simulink model "ACC_Model"  (Simulink 7.6)
settings: Solver=ode5  StartTime=0.0  StopTime=inf  FixedStep=1/100  RelTol=1e-3
undefined symbols (not defined in the file or in its folder): DiscIntNeverNeededParam
libraries: simulink x21, simulink_extras x6
(part 3 of 4)

== system ACC_Model/ACC_System/TIS2 Bend Road/TIS2 Sorting Fun ==
  note: === TIS1 Sorting Fun block ===
      |
      |  - transforms information from the first sensor
      |    to the more appropriate form.
  TIS2range [m] : Inport
  TIS2rangedot [m/s] : Inport  Port=2
  TIS2theta [deg] : Inport  Port=3
  Degrees to Radians : simulink_extras/Transformations/Degrees to Radians  SystemSampleTime=-1
  Switch : Switch  Criteria=u2 ~= 0
  Unary Minus : UnaryMinus
  Unary Minus1 : UnaryMinus
  range max : Constant  Value=5*TISMaxRange(2)
  TIS2_RANGE [m] : Outport
  TIS2_RANGEDOT [m/s] : Outport  Port=2
  TIS2_THETA [rad] : Outport  Port=3
  wires:
  Unary Minus/1 -> Degrees to Radians/1
  Switch/1 -> TIS2_RANGE [m]/1
  TIS2rangedot [m/s]/1 -> Unary Minus1/1
  range max/1 -> Switch/3
  Degrees to Radians/1 -> TIS2_THETA [rad]/1
  TIS2range [m]/1 -> Switch/2, Switch/1
  TIS2theta [deg]/1 -> Unary Minus/1
  Unary Minus1/1 -> TIS2_RANGEDOT [m/s]/1

== system ACC_Model/ACC_System/TIS2 Straight Road/Hold ==
  HWTflagIN : Inport
  lead_vel_in : Inport  Port=2
  HWTflagIN1 : InportShadow  Port=1
  If : If  IfExpression=u1 < 0.1  SampleTime=Tsensor
  If Action Subsystem : Subsystem  TreatAsAtomicUnit=on
  If Action Subsystem1 : Subsystem  TreatAsAtomicUnit=on
  Merge : Merge
  HWT_flag : Outport
  wires:
  lead_vel_in/1 -> If/1
  If/1 -> If Action Subsystem/Action
  If/2 -> If Action Subsystem1/Action
  If Action Subsystem/1(Out1) -> Merge/1
  If Action Subsystem1/1(Out1) -> Merge/2
  Merge/1 -> HWT_flag/1
  HWTflagIN/1 -> If Action Subsystem1/1(In1)
  HWTflagIN1/1 -> If Action Subsystem/1(In1)

== system ACC_Model/ACC_System/TIS2 Straight Road/TIS2 Closest Object ==
  note: === TIS2 Closest Object block ===
      |
      |  - passing through data about potentially the most dangerous object driving on the straight road.
  TIS2_rangedot [m/s] : Inport
  TIS2_distance [m] : Inport  Port=2
  index : Inport  Port=3
  Selector1 : Selector  InputPortWidth=TISdet(2)  IndexOptions=Index vector (port)  Indices=[1 3]  OutputSizes=1
  Selector2 : Selector  InputPortWidth=TISdet(2)  IndexOptions=Index vector (port)  Indices=[1 3]  OutputSizes=1
  rangedot [m/s] : Outport
  distance [m/s] : Outport  Port=2
  wires:
  Selector2/1 -> distance [m/s]/1
  TIS2_distance [m]/1 -> Selector2/1
  Selector1/1 -> rangedot [m/s]/1
  TIS2_rangedot [m/s]/1 -> Selector1/1
  index/1 -> Selector1/2, Selector2/2

== system ACC_Model/ACC_System/TIS2 Straight Road/TIS2 HWT Computing ==
  note: === TIS1 HWT Computing block===
      |
      |  - computes HeadWay Time (HWT) as it is defined in ISO norms.
  Distance [m] : Inport
  HWT demanded : Inport  Port=2
  Velocity [m/s] : Inport  Port=3
  If : If
  If Action Subsystem : Subsystem  TreatAsAtomicUnit=on
  If Action Subsystem1 : Subsystem  TreatAsAtomicUnit=on
  Merge : Merge
  HWT [s] : Outport
  wires:
  Velocity [m/s]/1 -> If/1, If Action Subsystem/2(Velocity [m/s])
  If/1 -> If Action Subsystem/Action
  If/2 -> If Action Subsystem1/Action
  If Action Subsystem/1(HWT [s]) -> Merge/1
  If Action Subsystem1/1(Out1) -> Merge/2
  Merge/1 -> HWT [s]/1
  Distance [m]/1 -> If Action Subsystem/1(Distance [m])
  HWT demanded/1 -> If Action Subsystem1/1(HWT demanded [s])

== system ACC_Model/ACC_System/TIS2 Straight Road/TIS2 HWT Computing2 ==
  note: === TIS1 HWT Computing block===
      |
      |  - computes HeadWay Time (HWT) as it is defined in ISO norms.
  Distance [m] : Inport
  Velocity [m/s] : Inport  Port=2
  If : If
  If Action Subsystem : Subsystem  TreatAsAtomicUnit=on
  If Action Subsystem1 : Subsystem  TreatAsAtomicUnit=on
  Merge : Merge
  HWT [s] : Outport
  wires:
  Velocity [m/s]/1 -> If/1, If Action Subsystem/2(Velocity [m/s])
  If/1 -> If Action Subsystem/Action
  If/2 -> If Action Subsystem1/Action
  If Action Subsystem/1(HWT [s]) -> Merge/1
  If Action Subsystem1/1(Out1) -> Merge/2
  Merge/1 -> HWT [s]/1
  Distance [m]/1 -> If Action Subsystem/1(Distance [m])

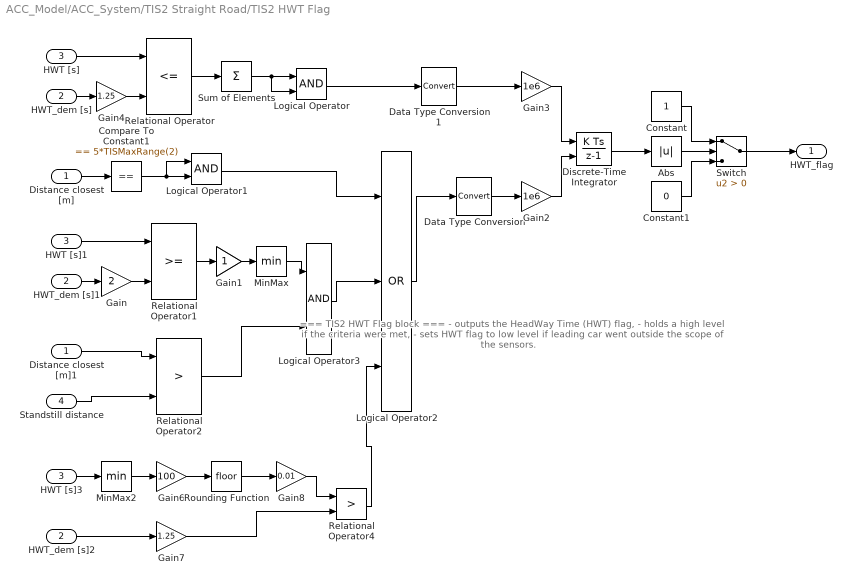
== system ACC_Model/ACC_System/TIS2 Straight Road/TIS2 HWT Flag ==
  note: === TIS2 HWT Flag block ===
      |
      |  - outputs the HeadWay Time (HWT) flag,
      |  - holds a high level if the criteria were met,
      |  - sets HWT flag to low level if leading car
      |    went outside the scope of the sensors.
  Distance closest [m] : Inport
  HWT_dem [s] : Inport  Port=2
  HWT [s] : Inport  Port=3
  Standstill distance : Inport  Port=4
  Abs : Abs
  Compare To Constant1 : simulink/Logic and Bit Operations/Compare To Constant  SystemSampleTime=-1  relop===  const=5*TISMaxRange(2)  LogicOutDataTypeMode=uint8
  Constant : Constant
  Constant1 : Constant  Value=0
  Data Type Conversion : DataTypeConversion
  Data Type Conversion1 : DataTypeConversion
  Discrete-Time Integrator : DiscreteIntegrator  ExternalReset=level  SampleTime=Tsensor  ICPrevOutput=DiscIntNeverNeededParam  ICPrevScaledInput=DiscIntNeverNeededParam
  Distance closest [m]1 : InportShadow  Port=1
  Gain : Gain  Gain=2
  Gain1 : Gain
  Gain2 : Gain  Gain=1e6  OutDataTypeStr=double
  Gain3 : Gain  Gain=1e6  OutDataTypeStr=double
  Gain4 : Gain  Gain=1.25
  Gain6 : Gain  Gain=100
  Gain7 : Gain  Gain=1.25
  Gain8 : Gain  Gain=0.01
  HWT [s]1 : InportShadow  Port=3
  HWT [s]3 : InportShadow  Port=3
  HWT_dem [s]1 : InportShadow  Port=2
  HWT_dem [s]2 : InportShadow  Port=2
  Logical Operator : Logic  AllPortsSameDT=off  OutDataTypeStr=boolean
  Logical Operator1 : Logic  AllPortsSameDT=off  OutDataTypeStr=boolean
  Logical Operator2 : Logic  Operator=OR  Inputs=3  AllPortsSameDT=off  OutDataTypeStr=boolean
  Logical Operator3 : Logic  AllPortsSameDT=off  OutDataTypeStr=boolean
  MinMax : MinMax
  MinMax2 : MinMax
  Relational Operator : RelationalOperator  Operator=<=  OutDataTypeStr=boolean
  Relational Operator1 : RelationalOperator  OutDataTypeStr=boolean
  Relational Operator2 : RelationalOperator  Operator=>  OutDataTypeStr=boolean
  Relational Operator4 : RelationalOperator  Operator=>  OutDataTypeStr=boolean
  Rounding Function : Rounding
  Sum of Elements : Sum  Inputs=+
  Switch : Switch  Criteria=u2 > Threshold
  HWT_flag : Outport
  wires:
  Logical Operator1/1 -> Logical Operator2/1
  Distance closest [m]/1 -> Compare To Constant1/1
  Logical Operator/1 -> Data Type Conversion1/1
  Sum of Elements/1 -> Logical Operator/2, Logical Operator/1
  Relational Operator/1 -> Sum of Elements/1
  HWT_dem [s]/1 -> Gain4/1
  HWT [s]/1 -> Relational Operator/1
  Compare To Constant1/1 -> Logical Operator1/2, Logical Operator1/1
  HWT [s]1/1 -> Relational Operator1/1
  Gain/1 -> Relational Operator1/2
  Relational Operator1/1 -> Gain1/1
  Gain1/1 -> MinMax/1
  Logical Operator2/1 -> Data Type Conversion/1
  HWT_dem [s]1/1 -> Gain/1
  Distance closest [m]1/1 -> Relational Operator2/1
  Standstill distance/1 -> Relational Operator2/2
  Relational Operator2/1 -> Logical Operator3/2
  MinMax/1 -> Logical Operator3/1
  Logical Operator3/1 -> Logical Operator2/2
  Gain2/1 -> Discrete-Time Integrator/2
  Gain3/1 -> Discrete-Time Integrator/1
  Discrete-Time Integrator/1 -> Abs/1
  Abs/1 -> Switch/2
  Constant/1 -> Switch/1
  Constant1/1 -> Switch/3
  Switch/1 -> HWT_flag/1
  Gain4/1 -> Relational Operator/2
  HWT_dem [s]2/1 -> Gain7/1
  HWT [s]3/1 -> MinMax2/1
  Gain6/1 -> Rounding Function/1
  Rounding Function/1 -> Gain8/1
  MinMax2/1 -> Gain6/1
  Gain8/1 -> Relational Operator4/1
  Gain7/1 -> Relational Operator4/2
  Relational Operator4/1 -> Logical Operator2/3
  Data Type Conversion/1 -> Gain2/1
  Data Type Conversion1/1 -> Gain3/1

== system ACC_Model/ACC_System/TIS2 Straight Road/TIS2 Lead Car Longitudinal Velocity ==
  note: === TIS2 Lead Car Longitudinal Velocity block ===
      |
      |  - computes the leading car absolute velocity and safe distance between the EGO and leading car.
  HWT_dem (s) : Inport
  TIS2 Rangedot [m/s] : Inport  Port=2
  EGO Velocity [m/s] : Inport  Port=3
  Standstill [m] : Inport  Port=4
  Abs : Abs
  Add : Sum  Inputs=+-
  Constant : Constant  Value=0
  Divide : Product  Inputs=*/
  HWT_dem (s)1 : InportShadow  Port=1
  Product : Product  RndMeth=Zero
  Relational Operator : RelationalOperator  Operator=<=  OutDataTypeStr=boolean
  Switch : Switch  Criteria=u2 > Threshold
  Switch1 : Switch  Criteria=u2 ~= 0
  TIS2 Rangedot [m/s]1 : InportShadow  Port=2
  Safe distance [m] : Outport
  Lead velocity [m/s] : Outport  Port=2
  wires:
  Relational Operator/1 -> Switch/2
  Divide/1 -> Relational Operator/2
  HWT_dem (s)1/1 -> Divide/2
  Standstill [m]/1 -> Switch/1, Divide/1
  Switch/1 -> Safe distance [m]/1
  Product/1 -> Switch/3
  HWT_dem (s)/1 -> Product/2
  Add/1 -> Abs/1
  TIS2 Rangedot [m/s]/1 -> Add/2
  EGO Velocity [m/s]/1 -> Add/1
  Constant/1 -> Switch1/3
  Switch1/1 -> Lead velocity [m/s]/1
  TIS2 Rangedot [m/s]1/1 -> Switch1/2
  Abs/1 -> Product/1, Relational Operator/1, Switch1/1

== system ACC_Model/ACC_System/TIS2 Straight Road/TIS2 Objects On Lane ==
  note: === TIS2 Objects On Lane block ===
      |
      |  - decides which objects are on the same lane as the EGO car,
      |    when the EGO car drives straight.
  TIS2_range [m] : Inport
  TIS2_rangedot [m/s] : Inport  Port=2
  TIS2_theta [rad] : Inport  Port=3
  Abs : Abs
  Compare To Constant : simulink/Logic and Bit Operations/Compare To Constant  SystemSampleTime=-1  relop=<  const=LaneWidth/2  LogicOutDataTypeMode=boolean
  Constant : Constant  Value=0
  Product : Product  RndMeth=Zero
  Product1 : Product  RndMeth=Zero
  Switch1 : Switch  Criteria=u2 > Threshold  Threshold=0.5
  Switch3 : Switch  Criteria=u2 > Threshold  Threshold=0.5
  TIS2 range max (higher value) : Constant  Value=5*TISMaxRange(2)
  Trigonometric Function : Trigonometry
  Trigonometric Function1 : Trigonometry  Operator=cos
  TIS2_RANGEDOT [m/s] : Outport
  TIS2_Distance [m] : Outport  Port=2
  wires:
  Compare To Constant/1 -> Switch1/2, Switch3/2
  Constant/1 -> Switch1/3
  TIS2 range max (higher value)/1 -> Switch3/3
  Product1/1 -> Switch3/1
  Trigonometric Function1/1 -> Product1/2
  Abs/1 -> Trigonometric Function/1
  Switch3/1 -> TIS2_Distance [m]/1
  Switch1/1 -> TIS2_RANGEDOT [m/s]/1
  TIS2_rangedot [m/s]/1 -> Switch1/1
  TIS2_range [m]/1 -> Product/1, Product1/1
  Product/1 -> Compare To Constant/1
  Trigonometric Function/1 -> Product/2
  TIS2_theta [rad]/1 -> Trigonometric Function1/1, Abs/1

== system ACC_Model/ACC_System/TIS2 Straight Road/TIS2 Sorting Fun ==
  note: === TIS2 Sorting Fun block ===
      |
      |  - transforms information from the second sensor
      |    to the more appropriate form.
  TIS2range [m] : Inport
  TIS2rangedot [m/s] : Inport  Port=2
  TIS2theta [deg] : Inport  Port=3
  Degrees to Radians : simulink_extras/Transformations/Degrees to Radians  SystemSampleTime=-1
  Switch : Switch  Criteria=u2 ~= 0
  Unary Minus : UnaryMinus
  Unary Minus1 : UnaryMinus
  range max (higher value which  will not generate  high level of HWT flag) : Constant  Value=5*TISMaxRange(2)
  TIS2_RANGE [m] : Outport
  TIS2_RANGEDOT [m/s] : Outport  Port=2
  TIS2_THETA [rad] : Outport  Port=3
  wires:
  Unary Minus1/1 -> TIS2_RANGEDOT [m/s]/1
  TIS2theta [deg]/1 -> Unary Minus/1
  TIS2range [m]/1 -> Switch/2, Switch/1
  Degrees to Radians/1 -> TIS2_THETA [rad]/1
  range max (higher value which  will not generate  high level of HWT flag)/1 -> Switch/3
  TIS2rangedot [m/s]/1 -> Unary Minus1/1
  Switch/1 -> TIS2_RANGE [m]/1
  Unary Minus/1 -> Degrees to Radians/1

== system ACC_Model/ACC_System/TIS1 ACC action/If Action Subsystem/If Action Subsystem ==
  e : Inport
  th_in : Inport  Port=2
  Action Port : ActionPort  PropagateVarSize=During execution  ActionType=then
  Add : Sum  Inputs=+-
  Constant : Constant  Value=0
  Saturation : Saturate  UpperLimit=100  LowerLimit=0
  Subsystem : Subsystem
  Switch : Switch
  brake : Outport  InitialOutput=0
  throttle : Outport  Port=2  InitialOutput=0
  wires:
  Subsystem/1(out) -> Switch/1, Add/2
  e/1 -> Subsystem/1(e)
  Saturation/1 -> throttle/1
  Constant/1 -> brake/1
  th_in/1 -> Switch/3, Add/1
  Add/1 -> Switch/2
  Switch/1 -> Saturation/1

== system ACC_Model/ACC_System/TIS1 ACC action/If Action Subsystem/If Action Subsystem1 ==
  rd : Inport
  e : Inport  Port=2
  Vp : Inport  Port=3
  EGO distance : Inport  Port=4
  HWT_dem : Inport  Port=5
  th_in : Inport  Port=6
  Action Port : ActionPort  PropagateVarSize=During execution  ActionType=else
  Add : Sum  Inputs=+-
  Constant : Constant  Value=drd/3.6
  If : If  SampleTime=Tsensor
  If Action Subsystem : Subsystem  TreatAsAtomicUnit=on
  If Action Subsystem1 : Subsystem  TreatAsAtomicUnit=on
  Merge : Merge
  Merge1 : Merge
  dec : Outport  InitialOutput=0
  throttle : Outport  Port=2  InitialOutput=0
  wires:
  rd/1 -> Add/1, If Action Subsystem/1(rd), If Action Subsystem1/1(rd)
  Constant/1 -> Add/2
  Add/1 -> If/1
  If/1 -> If Action Subsystem/Action
  If/2 -> If Action Subsystem1/Action
  e/1 -> If Action Subsystem/2(e [m]), If Action Subsystem1/2(e [m]), If Action Subsystem1/6(e_acc)
  If Action Subsystem/1(deceleration_[m/s2]) -> Merge/1
  If Action Subsystem/2(throttle) -> Merge1/1
  Merge/1 -> dec/1
  Merge1/1 -> throttle/1
  If Action Subsystem1/2(brake) -> Merge/2
  If Action Subsystem1/1(throttle) -> Merge1/2
  EGO distance/1 -> If Action Subsystem1/3(EGO_distance[m])
  HWT_dem/1 -> If Action Subsystem1/4(HWT_dem)
  Vp/1 -> If Action Subsystem1/5(Vp)
  th_in/1 -> If Action Subsystem1/7(th_in)

== system ACC_Model/ACC_System/TIS1 ACC action/If Action Subsystem1/If Action Subsystem ==
  Action Port : ActionPort  PropagateVarSize=During execution  ActionType=then
  Constant : Constant  Value=0
  Constant1 : Constant  Value=0
  dec : Outport  InitialOutput=0
  throttle : Outport  Port=2  InitialOutput=0
  wires:
  Constant/1 -> dec/1
  Constant1/1 -> throttle/1

== system ACC_Model/ACC_System/TIS1 ACC action/If Action Subsystem1/If Action Subsystem1 ==
  rd : Inport
  e : Inport  Port=2
  Vp : Inport  Port=3
  Ego distance : Inport  Port=4
  HWT dem : Inport  Port=5
  Action Port : ActionPort  PropagateVarSize=During execution  ActionType=else
  Add : Sum  Inputs=+-
  Constant : Constant  Value=drd/3.6
  If : If  SampleTime=Tsensor
  If Action Subsystem : Subsystem  TreatAsAtomicUnit=on
  If Action Subsystem1 : Subsystem  TreatAsAtomicUnit=on
  Merge : Merge
  Merge1 : Merge
  dec : Outport  InitialOutput=0
  throttle : Outport  Port=2  InitialOutput=0
  wires:
  rd/1 -> Add/1, If Action Subsystem1/1(rd)
  Constant/1 -> Add/2
  Add/1 -> If/1
  If/1 -> If Action Subsystem/Action
  If/2 -> If Action Subsystem1/Action
  e/1 -> If Action Subsystem1/2(e [m])
  Vp/1 -> If Action Subsystem1/5(Vp)
  If Action Subsystem/1(dec) -> Merge/1
  If Action Subsystem/2(throttle) -> Merge1/1
  Merge/1 -> dec/1
  Merge1/1 -> throttle/1
  If Action Subsystem1/2(brake) -> Merge/2
  If Action Subsystem1/1(throttle) -> Merge1/2
  Ego distance/1 -> If Action Subsystem1/3(EGO_distance[m])
  HWT dem/1 -> If Action Subsystem1/4(HWT_dem)

== system ACC_Model/ACC_System/TIS1 Bend Road/Hold/If Action Subsystem ==
  In1 : Inport
  Action Port : ActionPort  InitializeStates=reset  PropagateVarSize=During execution  ActionType=then
  Constant : Constant
  Constant1 : Constant  Value=0
  Discrete-Time Integrator : DiscreteIntegrator  gainval=100  InitialConditionSource=external  InitialConditionMode=State only (most efficient)  SampleTime=Tsensor  LimitOutput=on  UpperSaturationLimit=1  LowerSaturationLimit=0  ICPrevOutput=DiscIntNeverNeededParam  ICPrevScaledInput=DiscIntNeverNeededParam
  Gain3 : Gain  Gain=1e6  OutDataTypeStr=double
  Switch : Switch  Criteria=u2 > Threshold
  Out1 : Outport
  wires:
  Gain3/1 -> Discrete-Time Integrator/1
  In1/1 -> Gain3/1, Switch/2
  Discrete-Time Integrator/1 -> Out1/1
  Switch/1 -> Discrete-Time Integrator/2
  Constant/1 -> Switch/1
  Constant1/1 -> Switch/3

== system ACC_Model/ACC_System/TIS1 Bend Road/Hold/If Action Subsystem1 ==
  In1 : Inport
  Action Port : ActionPort  PropagateVarSize=During execution  ActionType=else
  Out1 : Outport
  wires:
  In1/1 -> Out1/1

== system ACC_Model/ACC_System/TIS1 Bend Road/TIS1 HWT Computing/If Action Subsystem ==
  Distance [m] : Inport
  Velocity [m/s] : Inport  Port=2
  Action Port : ActionPort  PropagateVarSize=During execution  ActionType=then
  Product : Product  Inputs=*/  RndMeth=Zero
  HWT [s] : Outport
  wires:
  Distance [m]/1 -> Product/1
  Velocity [m/s]/1 -> Product/2
  Product/1 -> HWT [s]/1

== system ACC_Model/ACC_System/TIS1 Bend Road/TIS1 HWT Computing/If Action Subsystem1 ==
  Action Port : ActionPort  PropagateVarSize=During execution  ActionType=else
  Constant : Constant  Value=inf
  Out1 : Outport  InitialOutput=0
  wires:
  Constant/1 -> Out1/1

== system ACC_Model/ACC_System/TIS1 Straight Road/Hold/If Action Subsystem ==
  In1 : Inport
  Action Port : ActionPort  InitializeStates=reset  PropagateVarSize=During execution  ActionType=then
  Constant : Constant
  Constant1 : Constant  Value=0
  Discrete-Time Integrator : DiscreteIntegrator  gainval=100  InitialConditionSource=external  InitialConditionMode=State only (most efficient)  SampleTime=Tsensor  LimitOutput=on  UpperSaturationLimit=1  LowerSaturationLimit=0  ICPrevOutput=DiscIntNeverNeededParam  ICPrevScaledInput=DiscIntNeverNeededParam
  Gain3 : Gain  Gain=1e6  OutDataTypeStr=double
  Switch : Switch  Criteria=u2 > Threshold
  Out1 : Outport
  wires:
  Gain3/1 -> Discrete-Time Integrator/1
  In1/1 -> Gain3/1, Switch/2
  Discrete-Time Integrator/1 -> Out1/1
  Switch/1 -> Discrete-Time Integrator/2
  Constant/1 -> Switch/1
  Constant1/1 -> Switch/3

== system ACC_Model/ACC_System/TIS1 Straight Road/Hold/If Action Subsystem1 ==
  In1 : Inport
  Action Port : ActionPort  PropagateVarSize=During execution  ActionType=else
  Out1 : Outport
  wires:
  In1/1 -> Out1/1

== system ACC_Model/ACC_System/TIS1 Straight Road/TIS1 HWT Computing/If Action Subsystem ==
  Distance [m] : Inport
  Velocity [m/s] : Inport  Port=2
  Action Port : ActionPort  PropagateVarSize=During execution  ActionType=then
  Product : Product  Inputs=*/  RndMeth=Zero
  HWT [s] : Outport
  wires:
  Distance [m]/1 -> Product/1
  Velocity [m/s]/1 -> Product/2
  Product/1 -> HWT [s]/1

== system ACC_Model/ACC_System/TIS1 Straight Road/TIS1 HWT Computing/If Action Subsystem1 ==
  HWT demanded [s] : Inport
  Action Port : ActionPort  PropagateVarSize=During execution  ActionType=else
  Gain : Gain  Gain=2*ones(TISdet(1),1)
  Out1 : Outport
  wires:
  Gain/1 -> Out1/1
  HWT demanded [s]/1 -> Gain/1

== system ACC_Model/ACC_System/TIS1 Straight Road/TIS1 HWT Computing1/If Action Subsystem ==
  Distance [m] : Inport
  Velocity [m/s] : Inport  Port=2
  Action Port : ActionPort  PropagateVarSize=During execution  ActionType=then
  Product : Product  Inputs=*/  RndMeth=Zero
  HWT [s] : Outport
  wires:
  Distance [m]/1 -> Product/1
  Velocity [m/s]/1 -> Product/2
  Product/1 -> HWT [s]/1

== system ACC_Model/ACC_System/TIS1 Straight Road/TIS1 HWT Computing1/If Action Subsystem1 ==
  Action Port : ActionPort  PropagateVarSize=During execution  ActionType=else
  Constant : Constant  Value=inf
  Out1 : Outport  InitialOutput=0
  wires:
  Constant/1 -> Out1/1

== system ACC_Model/ACC_System/TIS2 ACC action/If Action Subsystem/If Action Subsystem ==
  e : Inport
  th_in : Inport  Port=2
  Action Port : ActionPort  PropagateVarSize=During execution  ActionType=then
  Add : Sum  Inputs=+-
  Constant : Constant  Value=0
  Rate Limiter : RateLimiter  RisingSlewLimit=BrakeMax*1e3  FallingSlewLimit=-BrakeMax*1e3  SampleTimeMode=inherited
  Saturation : Saturate  UpperLimit=100  LowerLimit=0
  Subsystem : Subsystem
  Switch : Switch
  brake : Outport  InitialOutput=0
  throttle : Outport  Port=2  InitialOutput=0
  wires:
  Subsystem/1(out) -> Add/2, Switch/1
  e/1 -> Subsystem/1(e)
  Saturation/1 -> Rate Limiter/1
  Constant/1 -> brake/1
  Rate Limiter/1 -> throttle/1
  th_in/1 -> Add/1, Switch/3
  Add/1 -> Switch/2
  Switch/1 -> Saturation/1

== system ACC_Model/ACC_System/TIS2 ACC action/If Action Subsystem/If Action Subsystem1 ==
  rd : Inport
  e : Inport  Port=2
  Vp : Inport  Port=3
  EGO distance : Inport  Port=4
  HWT_dem : Inport  Port=5
  th_in : Inport  Port=6
  Action Port : ActionPort  PropagateVarSize=During execution  ActionType=else
  Add : Sum  Inputs=+-
  Constant : Constant  Value=drd/3.6
  If : If
  If Action Subsystem : Subsystem  TreatAsAtomicUnit=on
  If Action Subsystem1 : Subsystem  TreatAsAtomicUnit=on
  Merge : Merge
  Merge1 : Merge
  dec : Outport  InitialOutput=0
  throttle : Outport  Port=2  InitialOutput=0
  wires:
  rd/1 -> Add/1, If Action Subsystem/1(rd), If Action Subsystem1/1(rd)
  Constant/1 -> Add/2
  Add/1 -> If/1
  If/1 -> If Action Subsystem/Action
  If/2 -> If Action Subsystem1/Action
  e/1 -> If Action Subsystem/2(e [m]), If Action Subsystem1/2(e [m]), If Action Subsystem1/6(e_acc)
  If Action Subsystem/1(deceleration_[m/s2]) -> Merge/1
  If Action Subsystem/2(throttle) -> Merge1/1
  Merge/1 -> dec/1
  Merge1/1 -> throttle/1
  If Action Subsystem1/2(brake) -> Merge/2
  If Action Subsystem1/1(throttle) -> Merge1/2
  EGO distance/1 -> If Action Subsystem1/3(EGO_distance[m])
  HWT_dem/1 -> If Action Subsystem1/4(HWT_dem)
  Vp/1 -> If Action Subsystem1/5(Vp)
  th_in/1 -> If Action Subsystem1/7(th_in)

== system ACC_Model/ACC_System/TIS2 ACC action/If Action Subsystem1/If Action Subsystem ==
  Action Port : ActionPort  PropagateVarSize=During execution  ActionType=then
  Constant : Constant  Value=0
  Constant1 : Constant  Value=0
  dec : Outport  InitialOutput=0
  throttle : Outport  Port=2  InitialOutput=0
  wires:
  Constant/1 -> dec/1
  Constant1/1 -> throttle/1

== system ACC_Model/ACC_System/TIS2 ACC action/If Action Subsystem1/If Action Subsystem1 ==
  rd : Inport
  e : Inport  Port=2
  Vp : Inport  Port=3
  Ego distance : Inport  Port=4
  HWT dem : Inport  Port=5
  Action Port : ActionPort  PropagateVarSize=During execution  ActionType=else
  Add : Sum  Inputs=+-
  Constant : Constant  Value=drd/3.6
  If : If
  If Action Subsystem : Subsystem  TreatAsAtomicUnit=on
  If Action Subsystem1 : Subsystem  TreatAsAtomicUnit=on
  Merge : Merge
  Merge1 : Merge
  dec : Outport  InitialOutput=0
  throttle : Outport  Port=2  InitialOutput=0
  wires:
  rd/1 -> Add/1, If Action Subsystem1/1(rd)
  Constant/1 -> Add/2
  Add/1 -> If/1
  If/1 -> If Action Subsystem/Action
  If/2 -> If Action Subsystem1/Action
  e/1 -> If Action Subsystem1/2(e [m])
  Vp/1 -> If Action Subsystem1/5(Vp)
  If Action Subsystem/1(dec) -> Merge/1
  If Action Subsystem/2(throttle) -> Merge1/1
  Merge/1 -> dec/1
  Merge1/1 -> throttle/1
  If Action Subsystem1/2(brake) -> Merge/2
  If Action Subsystem1/1(throttle) -> Merge1/2
  Ego distance/1 -> If Action Subsystem1/3(EGO_distance[m])
  HWT dem/1 -> If Action Subsystem1/4(HWT_dem)

== system ACC_Model/ACC_System/TIS2 ACC action/Stop & Go/If Action Subsystem ==
  TIS2_Distance[m] : Inport
  TIS2_Safe_Distance [m] : Inport  Port=2
  rd : Inport  Port=3
  th_in : Inport  Port=4
  Vp : Inport  Port=5
  Stand : Inport  Port=6
  Action Port : ActionPort  PropagateVarSize=During execution  ActionType=then
  Add2 : Sum  Inputs=-+
  If : If
  If Action Subsystem : Subsystem  TreatAsAtomicUnit=on
  If Action Subsystem1 : Subsystem  TreatAsAtomicUnit=on
  Merge : Merge
  Merge1 : Merge
  Stand1 : InportShadow  Port=6
  br : Outport
  th : Outport  Port=2
  wires:
  TIS2_Distance[m]/1 -> Add2/2, If Action Subsystem/4(dis), If Action Subsystem1/4(dis)
  TIS2_Safe_Distance [m]/1 -> Add2/1
  Add2/1 -> If/1, If Action Subsystem/2(e [m]), If Action Subsystem1/2(e [m])
  If/2 -> If Action Subsystem1/Action
  If/1 -> If Action Subsystem/Action
  rd/1 -> If Action Subsystem/1(rd), If Action Subsystem1/1(rd1)
  Merge1/1 -> th/1
  Merge/1 -> br/1
  If Action Subsystem/1(brake) -> Merge/1
  If Action Subsystem/2(throttle) -> Merge1/2
  If Action Subsystem1/1(brake) -> Merge/2
  If Action Subsystem1/2(throttle1) -> Merge1/1
  Vp/1 -> If Action Subsystem1/3(Vp)
  Stand/1 -> If Action Subsystem/5(Stand)
  Stand1/1 -> If Action Subsystem1/5(stand)
  th_in/1 -> If Action Subsystem/3(th_in)

== system ACC_Model/ACC_System/TIS2 ACC action/Stop & Go/If Action Subsystem1 ==
  In1 : Inport
  In2 : Inport  Port=2
  Action Port : ActionPort  PropagateVarSize=During execution  ActionType=else
  Out1 : Outport
  Out2 : Outport  Port=2
  wires:
  In1/1 -> Out1/1
  In2/1 -> Out2/1

== system ACC_Model/ACC_System/TIS2 ACC action/Stop & Go/Subsystem ==
  In1 : Inport
  In2 : Inport  Port=2
  EGO_Velocity [m/s] : Inport  Port=3
  Abs : Abs
  Abs1 : Abs
  Compare To Constant : simulink/Logic and Bit Operations/Compare To Constant  SystemSampleTime=-1  relop=<=  const=0.1  LogicOutDataTypeMode=uint8  ZeroCross=off
  Compare To Constant1 : simulink/Logic and Bit Operations/Compare To Constant  SystemSampleTime=-1  relop=<=  const=0.1  LogicOutDataTypeMode=uint8  ZeroCross=off
  Logical Operator1 : Logic  AllPortsSameDT=off  OutDataTypeStr=boolean
  Max Brake ON : Constant  Value=BrakeMax * J_xx / Qfac / Rw
  Switch1 : Switch  Criteria=u2 > Threshold
  BrakePres[bar] : Outport
  wires:
  In1/1 -> Abs/1
  EGO_Velocity [m/s]/1 -> Abs1/1
  Compare To Constant/1 -> Logical Operator1/1
  Compare To Constant1/1 -> Logical Operator1/2
  Logical Operator1/1 -> Switch1/2
  Max Brake ON/1 -> Switch1/1
  Switch1/1 -> BrakePres[bar]/1
  Abs/1 -> Compare To Constant/1
  Abs1/1 -> Compare To Constant1/1
  In2/1 -> Switch1/3

== system ACC_Model/ACC_System/TIS2 Bend Road/Hold/If Action Subsystem ==
  In1 : Inport
  Action Port : ActionPort  InitializeStates=reset  PropagateVarSize=During execution  ActionType=then
  Constant : Constant
  Constant1 : Constant  Value=0
  Discrete-Time Integrator : DiscreteIntegrator  gainval=100  InitialConditionSource=external  InitialConditionMode=State only (most efficient)  SampleTime=Tsensor  LimitOutput=on  UpperSaturationLimit=1  LowerSaturationLimit=0  ICPrevOutput=DiscIntNeverNeededParam  ICPrevScaledInput=DiscIntNeverNeededParam
  Gain3 : Gain  Gain=1e6  OutDataTypeStr=double
  Switch : Switch  Criteria=u2 > Threshold
  Out1 : Outport
  wires:
  Gain3/1 -> Discrete-Time Integrator/1
  In1/1 -> Gain3/1, Switch/2
  Discrete-Time Integrator/1 -> Out1/1
  Switch/1 -> Discrete-Time Integrator/2
  Constant/1 -> Switch/1
  Constant1/1 -> Switch/3

== system ACC_Model/ACC_System/TIS2 Bend Road/Hold/If Action Subsystem1 ==
  In1 : Inport
  Action Port : ActionPort  PropagateVarSize=During execution  ActionType=else
  Out1 : Outport
  wires:
  In1/1 -> Out1/1

== system ACC_Model/ACC_System/TIS2 Bend Road/TIS1 HWT Computing/If Action Subsystem ==
  Distance [m] : Inport
  Velocity [m/s] : Inport  Port=2
  Action Port : ActionPort  PropagateVarSize=During execution  ActionType=then
  Product : Product  Inputs=*/  RndMeth=Zero
  HWT [s] : Outport
  wires:
  Distance [m]/1 -> Product/1
  Velocity [m/s]/1 -> Product/2
  Product/1 -> HWT [s]/1

== system ACC_Model/ACC_System/TIS2 Bend Road/TIS1 HWT Computing/If Action Subsystem1 ==
  Action Port : ActionPort  PropagateVarSize=During execution  ActionType=else
  Constant : Constant  Value=inf
  Out1 : Outport  InitialOutput=0
  wires:
  Constant/1 -> Out1/1

== system ACC_Model/ACC_System/TIS2 Straight Road/Hold/If Action Subsystem ==
  In1 : Inport
  Action Port : ActionPort  InitializeStates=reset  PropagateVarSize=During execution  ActionType=then
  Constant : Constant
  Constant1 : Constant  Value=0
  Discrete-Time Integrator : DiscreteIntegrator  gainval=100  InitialConditionSource=external  InitialConditionMode=State only (most efficient)  SampleTime=Tsensor  LimitOutput=on  UpperSaturationLimit=1  LowerSaturationLimit=0  ICPrevOutput=DiscIntNeverNeededParam  ICPrevScaledInput=DiscIntNeverNeededParam
  Gain3 : Gain  Gain=1e6  OutDataTypeStr=double
  Switch : Switch  Criteria=u2 > Threshold
  Out1 : Outport
  wires:
  Gain3/1 -> Discrete-Time Integrator/1
  In1/1 -> Gain3/1, Switch/2
  Discrete-Time Integrator/1 -> Out1/1
  Switch/1 -> Discrete-Time Integrator/2
  Constant/1 -> Switch/1
  Constant1/1 -> Switch/3

== system ACC_Model/ACC_System/TIS2 Straight Road/Hold/If Action Subsystem1 ==
  In1 : Inport
  Action Port : ActionPort  PropagateVarSize=During execution  ActionType=else
  Out1 : Outport
  wires:
  In1/1 -> Out1/1

== system ACC_Model/ACC_System/TIS2 Straight Road/TIS2 HWT Computing/If Action Subsystem ==
  Distance [m] : Inport
  Velocity [m/s] : Inport  Port=2
  Action Port : ActionPort  PropagateVarSize=During execution  ActionType=then
  Product : Product  Inputs=*/  RndMeth=Zero
  HWT [s] : Outport
  wires:
  Distance [m]/1 -> Product/1
  Velocity [m/s]/1 -> Product/2
  Product/1 -> HWT [s]/1

== system ACC_Model/ACC_System/TIS2 Straight Road/TIS2 HWT Computing/If Action Subsystem1 ==
  HWT demanded [s] : Inport
  Action Port : ActionPort  PropagateVarSize=During execution  ActionType=else
  Gain : Gain  Gain=2*ones(TISdet(2),1)
  Out1 : Outport
  wires:
  Gain/1 -> Out1/1
  HWT demanded [s]/1 -> Gain/1

== system ACC_Model/ACC_System/TIS2 Straight Road/TIS2 HWT Computing2/If Action Subsystem ==
  Distance [m] : Inport
  Velocity [m/s] : Inport  Port=2
  Action Port : ActionPort  PropagateVarSize=During execution  ActionType=then
  Product : Product  Inputs=*/  RndMeth=Zero
  HWT [s] : Outport
  wires:
  Distance [m]/1 -> Product/1
  Velocity [m/s]/1 -> Product/2
  Product/1 -> HWT [s]/1

== system ACC_Model/ACC_System/TIS2 Straight Road/TIS2 HWT Computing2/If Action Subsystem1 ==
  Action Port : ActionPort  PropagateVarSize=During execution  ActionType=else
  Constant : Constant  Value=inf
  Out1 : Outport  InitialOutput=0
  wires:
  Constant/1 -> Out1/1

== system ACC_Model/ACC_System/TIS1 ACC action/If Action Subsystem/If Action Subsystem/Subsystem ==
  e : Inport
  Difference : simulink/Discrete/Difference  SystemSampleTime=-1  ICPrevInput=0.0  OutMin=[]  OutMax=[]  OutDataType=sfix(16)  OutScaling=2^-10  DoSatur=off
  Discrete-Time Integrator : DiscreteIntegrator  SampleTime=Tsensor  ICPrevOutput=DiscIntNeverNeededParam  ICPrevScaledInput=DiscIntNeverNeededParam
  Gain : Gain  Gain=100
  Gain1 : Gain  Gain=0.3
  Gain2 : Gain  Gain=3.065*0.01
  Sum : Sum  Inputs=+++
  out : Outport
  wires:
  e/1 -> Gain1/1, Gain/1, Gain2/1
  Gain1/1 -> Discrete-Time Integrator/1
  Gain2/1 -> Difference/1
  Gain/1 -> Sum/1
  Discrete-Time Integrator/1 -> Sum/2
  Difference/1 -> Sum/3
  Sum/1 -> out/1

== system ACC_Model/ACC_System/TIS1 ACC action/If Action Subsystem/If Action Subsystem1/If Action Subsystem ==
  rd : Inport
  e [m] : Inport  Port=2
  Action Port : ActionPort  PropagateVarSize=During execution  ActionType=then
  Abs : Abs
  Constant : Constant  Value=0
  Divide : Product  Inputs=*/
  Gain : Gain  Gain=0.5
  Math Function : Math  Operator=square  SaturateOnIntegerOverflow=on
  Saturation1 : Saturate  UpperLimit=inf  LowerLimit=0.02
  deceleration_[m/s2] : Outport  InitialOutput=0
  throttle : Outport  Port=2  InitialOutput=0
  wires:
  rd/1 -> Math Function/1
  Divide/1 -> Gain/1
  Math Function/1 -> Divide/1
  Abs/1 -> Saturation1/1
  Saturation1/1 -> Divide/2
  e [m]/1 -> Abs/1
  Gain/1 -> deceleration_[m/s2]/1
  Constant/1 -> throttle/1

== system ACC_Model/ACC_System/TIS1 ACC action/If Action Subsystem/If Action Subsystem1/If Action Subsystem1 ==
  rd : Inport
  e [m] : Inport  Port=2
  EGO_distance[m] : Inport  Port=3
  HWT_dem : Inport  Port=4
  Vp : Inport  Port=5
  e_acc : Inport  Port=6
  th_in : Inport  Port=7
  Action Port : ActionPort  PropagateVarSize=During execution  ActionType=else
  Add : Sum  Inputs=+-
  If : If  SampleTime=Tsensor
  If Action Subsystem : Subsystem  TreatAsAtomicUnit=on
  If Action Subsystem1 : Subsystem  TreatAsAtomicUnit=on
  Merge : Merge
  Merge1 : Merge
  Product : Product  RndMeth=Zero
  Vp1 : InportShadow  Port=5
  throttle : Outport  InitialOutput=0
  brake : Outport  Port=2  InitialOutput=0
  wires:
  HWT_dem/1 -> Product/1
  Vp1/1 -> Product/2
  EGO_distance[m]/1 -> Add/1
  Product/1 -> Add/2
  Add/1 -> If/1
  If/1 -> If Action Subsystem/Action
  If/2 -> If Action Subsystem1/Action
  rd/1 -> If Action Subsystem1/2(rd)
  e [m]/1 -> If Action Subsystem1/3(e [m])
  Vp/1 -> If Action Subsystem1/1(Vp)
  If Action Subsystem1/2(brake) -> Merge1/2
  If Action Subsystem1/1(throttle) -> Merge/2
  Merge1/1 -> brake/1
  Merge/1 -> throttle/1
  If Action Subsystem/1(brake) -> Merge1/1
  If Action Subsystem/2(throttle) -> Merge/1
  e_acc/1 -> If Action Subsystem/1(e)
  th_in/1 -> If Action Subsystem/2(th_in)

== system ACC_Model/ACC_System/TIS1 ACC action/If Action Subsystem1/If Action Subsystem1/If Action Subsystem ==
  Action Port : ActionPort  PropagateVarSize=During execution  ActionType=then
  Constant : Constant  Value=0
  Constant1 : Constant  Value=BrakeMax
  dec : Outport  InitialOutput=0
  throttle : Outport  Port=2  InitialOutput=0
  wires:
  Constant/1 -> throttle/1
  Constant1/1 -> dec/1

== system ACC_Model/ACC_System/TIS1 ACC action/If Action Subsystem1/If Action Subsystem1/If Action Subsystem1 ==
  rd : Inport
  e [m] : Inport  Port=2
  EGO_distance[m] : Inport  Port=3
  HWT_dem : Inport  Port=4
  Vp : Inport  Port=5
  Action Port : ActionPort  PropagateVarSize=During execution  ActionType=else
  Add : Sum  Inputs=+-
  If : If  SampleTime=Tsensor
  If Action Subsystem : Subsystem  TreatAsAtomicUnit=on
  If Action Subsystem1 : Subsystem  TreatAsAtomicUnit=on
  Merge : Merge
  Merge1 : Merge
  Product : Product  RndMeth=Zero
  Vp1 : InportShadow  Port=5
  throttle : Outport  InitialOutput=0
  brake : Outport  Port=2  InitialOutput=0
  wires:
  HWT_dem/1 -> Product/1
  Vp1/1 -> Product/2
  EGO_distance[m]/1 -> Add/1
  Product/1 -> Add/2
  Add/1 -> If/1
  If/1 -> If Action Subsystem/Action
  If/2 -> If Action Subsystem1/Action
  rd/1 -> If Action Subsystem1/2(rd)
  e [m]/1 -> If Action Subsystem1/3(e [m])
  Vp/1 -> If Action Subsystem1/1(Vp)
  Merge1/1 -> brake/1
  Merge/1 -> throttle/1
  If Action Subsystem/1(brake) -> Merge1/1
  If Action Subsystem/2(throttle) -> Merge/1
  If Action Subsystem1/2(brake) -> Merge1/2
  If Action Subsystem1/1(throttle) -> Merge/2

== system ACC_Model/ACC_System/TIS2 ACC action/If Action Subsystem/If Action Subsystem/Subsystem ==
  e : Inport
  Difference : simulink/Discrete/Difference  SystemSampleTime=-1  ICPrevInput=0.0  OutMin=[]  OutMax=[]  OutDataType=sfix(16)  OutScaling=2^-10  DoSatur=off
  Discrete-Time Integrator : DiscreteIntegrator  SampleTime=-1  ICPrevOutput=DiscIntNeverNeededParam  ICPrevScaledInput=DiscIntNeverNeededParam
  Gain : Gain  Gain=100
  Gain1 : Gain  Gain=0.3
  Gain2 : Gain  Gain=3.065*0.01
  Sum : Sum  Inputs=+++
  out : Outport
  wires:
  e/1 -> Gain1/1, Gain/1, Gain2/1
  Gain1/1 -> Discrete-Time Integrator/1
  Gain2/1 -> Difference/1
  Gain/1 -> Sum/1
  Discrete-Time Integrator/1 -> Sum/2
  Difference/1 -> Sum/3
  Sum/1 -> out/1

== system ACC_Model/ACC_System/TIS2 ACC action/If Action Subsystem/If Action Subsystem1/If Action Subsystem ==
  rd : Inport
  e [m] : Inport  Port=2
  Action Port : ActionPort  PropagateVarSize=During execution  ActionType=then
  Abs : Abs
  Constant : Constant  Value=0
  Divide : Product  Inputs=*/
  Gain : Gain  Gain=0.5
  Math Function : Math  Operator=square  SaturateOnIntegerOverflow=on
  Saturation1 : Saturate  UpperLimit=inf  LowerLimit=0.02
  deceleration_[m/s2] : Outport  InitialOutput=0
  throttle : Outport  Port=2  InitialOutput=0
  wires:
  rd/1 -> Math Function/1
  Divide/1 -> Gain/1
  Math Function/1 -> Divide/1
  Abs/1 -> Saturation1/1
  Saturation1/1 -> Divide/2
  e [m]/1 -> Abs/1
  Gain/1 -> deceleration_[m/s2]/1
  Constant/1 -> throttle/1

== system ACC_Model/ACC_System/TIS2 ACC action/If Action Subsystem/If Action Subsystem1/If Action Subsystem1 ==
  rd : Inport
  e [m] : Inport  Port=2
  EGO_distance[m] : Inport  Port=3
  HWT_dem : Inport  Port=4
  Vp : Inport  Port=5
  e_acc : Inport  Port=6
  th_in : Inport  Port=7
  Action Port : ActionPort  PropagateVarSize=During execution  ActionType=else
  Add : Sum  Inputs=+-
  If : If
  If Action Subsystem : Subsystem  TreatAsAtomicUnit=on
  If Action Subsystem1 : Subsystem  TreatAsAtomicUnit=on
  Merge : Merge
  Merge1 : Merge
  Product : Product  RndMeth=Zero
  Vp1 : InportShadow  Port=5
  throttle : Outport  InitialOutput=0
  brake : Outport  Port=2  InitialOutput=0
  wires:
  HWT_dem/1 -> Product/1
  Vp1/1 -> Product/2
  EGO_distance[m]/1 -> Add/1
  Product/1 -> Add/2
  Add/1 -> If/1
  If/1 -> If Action Subsystem/Action
  If/2 -> If Action Subsystem1/Action
  rd/1 -> If Action Subsystem1/2(rd)
  e [m]/1 -> If Action Subsystem1/3(e [m])
  Vp/1 -> If Action Subsystem1/1(Vp)
  If Action Subsystem1/2(brake) -> Merge1/2
  If Action Subsystem1/1(throttle) -> Merge/2
  Merge1/1 -> brake/1
  Merge/1 -> throttle/1
  If Action Subsystem/1(brake) -> Merge1/1
  If Action Subsystem/2(throttle) -> Merge/1
  e_acc/1 -> If Action Subsystem/1(e)
  th_in/1 -> If Action Subsystem/2(th_in)

== system ACC_Model/ACC_System/TIS2 ACC action/If Action Subsystem1/If Action Subsystem1/If Action Subsystem ==
  Action Port : ActionPort  PropagateVarSize=During execution  ActionType=then
  Constant : Constant  Value=0
  Constant1 : Constant  Value=BrakeMax
  dec : Outport  InitialOutput=0
  throttle : Outport  Port=2  InitialOutput=0
  wires:
  Constant/1 -> throttle/1
  Constant1/1 -> dec/1

== system ACC_Model/ACC_System/TIS2 ACC action/If Action Subsystem1/If Action Subsystem1/If Action Subsystem1 ==
  rd : Inport
  e [m] : Inport  Port=2
  EGO_distance[m] : Inport  Port=3
  HWT_dem : Inport  Port=4
  Vp : Inport  Port=5
  Action Port : ActionPort  PropagateVarSize=During execution  ActionType=else
  Add : Sum  Inputs=+-
  If : If
  If Action Subsystem : Subsystem  TreatAsAtomicUnit=on
  If Action Subsystem1 : Subsystem  TreatAsAtomicUnit=on
  Merge : Merge
  Merge1 : Merge
  Product : Product  RndMeth=Zero
  Vp1 : InportShadow  Port=5
  throttle : Outport  InitialOutput=0
  brake : Outport  Port=2  InitialOutput=0
  wires:
  HWT_dem/1 -> Product/1
  Vp1/1 -> Product/2
  EGO_distance[m]/1 -> Add/1
  Product/1 -> Add/2
  Add/1 -> If/1
  If/1 -> If Action Subsystem/Action
  If/2 -> If Action Subsystem1/Action
  rd/1 -> If Action Subsystem1/2(rd)
  e [m]/1 -> If Action Subsystem1/3(e [m])
  Vp/1 -> If Action Subsystem1/1(Vp)
  If Action Subsystem1/2(brake) -> Merge1/2
  If Action Subsystem1/1(throttle) -> Merge/2
  Merge1/1 -> brake/1
  Merge/1 -> throttle/1
  If Action Subsystem/1(brake) -> Merge1/1
  If Action Subsystem/2(throttle) -> Merge/1

== system ACC_Model/ACC_System/TIS2 ACC action/Stop & Go/If Action Subsystem/If Action Subsystem ==
  rd : Inport
  e [m] : Inport  Port=2
  th_in : Inport  Port=3
  dis : Inport  Port=4
  Stand : Inport  Port=5
  Action Port : ActionPort  PropagateVarSize=During execution  ActionType=then
  If : If
  If Action Subsystem : Subsystem  TreatAsAtomicUnit=on
  If Action Subsystem1 : Subsystem  TreatAsAtomicUnit=on
  Merge : Merge
  Merge1 : Merge
  brake : Outport  InitialOutput=0
  throttle : Outport  Port=2  InitialOutput=0
  wires:
  rd/1 -> If/1, If Action Subsystem/1(rd)
  If/1 -> If Action Subsystem/Action
  e [m]/1 -> If Action Subsystem/2(e [m]), If Action Subsystem1/1(e)
  If/2 -> If Action Subsystem1/Action
  If Action Subsystem/1(brake) -> Merge/1
  If Action Subsystem/2(throttle) -> Merge1/1
  Merge1/1 -> throttle/1
  Merge/1 -> brake/1
  If Action Subsystem1/1(brake) -> Merge/2
  If Action Subsystem1/2(throttle) -> Merge1/2
  th_in/1 -> If Action Subsystem1/2(th_in)
  dis/1 -> If Action Subsystem/3(dis)
  Stand/1 -> If Action Subsystem/4(stand)

== system ACC_Model/ACC_System/TIS2 ACC action/Stop & Go/If Action Subsystem/If Action Subsystem1 ==
  rd1 : Inport
  e [m] : Inport  Port=2
  Vp : Inport  Port=3
  dis : Inport  Port=4
  stand : Inport  Port=5
  Action Port : ActionPort  PropagateVarSize=During execution  ActionType=else
  Abs : Abs
  Add : Sum  Inputs=+-
  Bias : Bias  Bias=1
  Constant : Constant  Value=0
  Constant1 : Constant  Value=0
  Constant2 : Constant  Value=BrakeMax*J_xx/Qfac/Rw
  Constant3 : Constant  Value=BrakeMax*J_xx/Qfac/Rw
  Divide : Product  Inputs=*/
  Gain : Gain  Gain=0.5
  Gain1 : Gain  Gain=J_xx/Qfac/Rw
  Math Function : Math  Operator=square  SaturateOnIntegerOverflow=on
  Saturation : Saturate  UpperLimit=BrakeMax  LowerLimit=0
  Saturation1 : Saturate  UpperLimit=inf  LowerLimit=0.02
  Switch : Switch  Criteria=u2 > Threshold
  Switch1 : Switch  Criteria=u2 > Threshold  Threshold=1
  Switch2 : Switch  Criteria=u2 > Threshold
  rd2 : InportShadow  Port=1
  brake : Outport  InitialOutput=0
  throttle1 : Outport  Port=2  InitialOutput=0
  wires:
  rd1/1 -> Math Function/1
  Divide/1 -> Gain/1
  Math Function/1 -> Divide/1
  Abs/1 -> Saturation1/1
  Saturation1/1 -> Divide/2
  e [m]/1 -> Abs/1
  Constant/1 -> throttle1/1
  Saturation/1 -> Gain1/1
  Gain/1 -> Saturation/1
  rd2/1 -> Switch/2
  Gain1/1 -> Switch/1
  Constant1/1 -> Switch/3
  Vp/1 -> Switch1/2
  Switch/1 -> Switch1/1
  Constant2/1 -> Switch1/3
  dis/1 -> Bias/1
  stand/1 -> Add/2
  Add/1 -> Switch2/2
  Constant3/1 -> Switch2/3
  Bias/1 -> Add/1
  Switch2/1 -> brake/1
  Switch1/1 -> Switch2/1

== system ACC_Model/ACC_System/TIS1 ACC action/If Action Subsystem/If Action Subsystem1/If Action Subsystem1/If Action Subsystem ==
  e : Inport
  th_in : Inport  Port=2
  Action Port : ActionPort  PropagateVarSize=During execution  ActionType=then
  Constant : Constant  Value=0
  Constant1 : Constant  Value=0
  Rate Limiter : RateLimiter  RisingSlewLimit=BrakeMax*1e3  FallingSlewLimit=-BrakeMax*1e3  SampleTimeMode=inherited
  Saturation Dynamic : simulink/Discontinuities/Saturation Dynamic  SystemSampleTime=-1  OutMin=[]  OutMax=[]  OutDataTypeStr=Inherit: Same as second input  OutDataType=fixdt(1, 16)  OutScaling=2^-10  DoSatur=off
  Subsystem : Subsystem
  brake : Outport  InitialOutput=0
  throttle : Outport  Port=2  InitialOutput=0
  wires:
  Subsystem/1(out) -> Saturation Dynamic/2
  e/1 -> Subsystem/1(e)
  Saturation Dynamic/1 -> Rate Limiter/1
  Constant/1 -> brake/1
  Rate Limiter/1 -> throttle/1
  th_in/1 -> Saturation Dynamic/1
  Constant1/1 -> Saturation Dynamic/3

== system ACC_Model/ACC_System/TIS1 ACC action/If Action Subsystem/If Action Subsystem1/If Action Subsystem1/If Action Subsystem1 ==
  Vp : Inport
  rd : Inport  Port=2
  e [m] : Inport  Port=3
  Action Port : ActionPort  PropagateVarSize=During execution  ActionType=else
  Abs : Abs
  Constant1 : Constant  Value=0
  Constant2 : Constant  Value=LowSpeedActv
  Constant3 : Constant  Value=0
  Divide : Product  Inputs=*/
  Gain : Gain  Gain=3.6
  Gain1 : Gain  Gain=0.5
  Math Function : Math  Operator=square  SaturateOnIntegerOverflow=on
  Relational Operator : RelationalOperator  Operator=<  OutDataTypeStr=boolean
  Saturation1 : Saturate  UpperLimit=inf  LowerLimit=0.02
  Switch : Switch  Criteria=u2 > Threshold
  throttle : Outport  InitialOutput=0
  brake : Outport  Port=2  InitialOutput=0
  wires:
  Constant1/1 -> throttle/1
  Vp/1 -> Gain/1
  Gain/1 -> Relational Operator/1
  Constant2/1 -> Relational Operator/2
  Relational Operator/1 -> Switch/2
  Gain1/1 -> Switch/1
  Constant3/1 -> Switch/3
  rd/1 -> Math Function/1
  Divide/1 -> Gain1/1
  Math Function/1 -> Divide/1
  Abs/1 -> Saturation1/1
  Saturation1/1 -> Divide/2
  e [m]/1 -> Abs/1
  Switch/1 -> brake/1

== system ACC_Model/ACC_System/TIS1 ACC action/If Action Subsystem1/If Action Subsystem1/If Action Subsystem1/If Action Subsystem ==
  Action Port : ActionPort  PropagateVarSize=During execution  ActionType=then
  Constant : Constant  Value=0
  Constant1 : Constant  Value=0
  brake : Outport  InitialOutput=0
  throttle : Outport  Port=2  InitialOutput=0
  wires:
  Constant/1 -> brake/1
  Constant1/1 -> throttle/1

== system ACC_Model/ACC_System/TIS1 ACC action/If Action Subsystem1/If Action Subsystem1/If Action Subsystem1/If Action Subsystem1 ==
  Vp : Inport
  rd : Inport  Port=2
  e [m] : Inport  Port=3
  Action Port : ActionPort  PropagateVarSize=During execution  ActionType=else
  Abs : Abs
  Constant1 : Constant  Value=0
  Constant2 : Constant  Value=LowSpeedActv
  Constant3 : Constant  Value=0
  Divide : Product  Inputs=*/
  Gain : Gain  Gain=3.6
  Gain1 : Gain  Gain=0.5
  Math Function : Math  Operator=square  SaturateOnIntegerOverflow=on
  Relational Operator : RelationalOperator  Operator=<  OutDataTypeStr=boolean
  Saturation1 : Saturate  UpperLimit=inf  LowerLimit=0.02
  Switch : Switch  Criteria=u2 > Threshold
  throttle : Outport  InitialOutput=0
  brake : Outport  Port=2  InitialOutput=0
  wires:
  Constant1/1 -> throttle/1
  Vp/1 -> Gain/1
  Gain/1 -> Relational Operator/1
  Constant2/1 -> Relational Operator/2
  Relational Operator/1 -> Switch/2
  Gain1/1 -> Switch/1
  Constant3/1 -> Switch/3
  rd/1 -> Math Function/1
  Divide/1 -> Gain1/1
  Math Function/1 -> Divide/1
  Abs/1 -> Saturation1/1
  Saturation1/1 -> Divide/2
  e [m]/1 -> Abs/1
  Switch/1 -> brake/1

== system ACC_Model/ACC_System/TIS2 ACC action/If Action Subsystem/If Action Subsystem1/If Action Subsystem1/If Action Subsystem ==
  e : Inport
  th_in : Inport  Port=2
  Action Port : ActionPort  PropagateVarSize=During execution  ActionType=then
  Constant : Constant  Value=0
  Constant1 : Constant  Value=0
  Rate Limiter : RateLimiter  RisingSlewLimit=BrakeMax*1e3  FallingSlewLimit=-BrakeMax*1e3  SampleTimeMode=inherited
  Saturation Dynamic : simulink/Discontinuities/Saturation Dynamic  SystemSampleTime=-1  OutMin=[]  OutMax=[]  OutDataTypeStr=Inherit: Same as second input  OutDataType=fixdt(1, 16)  OutScaling=2^-10  DoSatur=off
  Subsystem : Subsystem
  brake : Outport  InitialOutput=0
  throttle : Outport  Port=2  InitialOutput=0
  wires:
  Subsystem/1(out) -> Saturation Dynamic/2
  e/1 -> Subsystem/1(e)
  Saturation Dynamic/1 -> Rate Limiter/1
  Constant/1 -> brake/1
  Rate Limiter/1 -> throttle/1
  th_in/1 -> Saturation Dynamic/1
  Constant1/1 -> Saturation Dynamic/3

== system ACC_Model/ACC_System/TIS2 ACC action/If Action Subsystem/If Action Subsystem1/If Action Subsystem1/If Action Subsystem1 ==
  Vp : Inport
  rd : Inport  Port=2
  e [m] : Inport  Port=3
  Action Port : ActionPort  PropagateVarSize=During execution  ActionType=else
  Abs : Abs
  Constant1 : Constant  Value=0
  Constant2 : Constant  Value=LowSpeedActv
  Constant3 : Constant  Value=0
  Divide : Product  Inputs=*/
  Gain : Gain  Gain=3.6
  Gain1 : Gain  Gain=0.5
  Math Function : Math  Operator=square  SaturateOnIntegerOverflow=on
  Relational Operator : RelationalOperator  Operator=<  OutDataTypeStr=boolean
  Saturation1 : Saturate  UpperLimit=inf  LowerLimit=0.02
  Switch : Switch  Criteria=u2 > Threshold
  throttle : Outport  InitialOutput=0
  brake : Outport  Port=2  InitialOutput=0
  wires:
  Constant1/1 -> throttle/1
  Vp/1 -> Gain/1
  Gain/1 -> Relational Operator/1
  Constant2/1 -> Relational Operator/2
  Relational Operator/1 -> Switch/2
  Gain1/1 -> Switch/1
  Constant3/1 -> Switch/3
  rd/1 -> Math Function/1
  Divide/1 -> Gain1/1
  Math Function/1 -> Divide/1
  Abs/1 -> Saturation1/1
  Saturation1/1 -> Divide/2
  e [m]/1 -> Abs/1
  Switch/1 -> brake/1

== system ACC_Model/ACC_System/TIS2 ACC action/If Action Subsystem1/If Action Subsystem1/If Action Subsystem1/If Action Subsystem ==
  Action Port : ActionPort  PropagateVarSize=During execution  ActionType=then
  Constant : Constant  Value=0
  Constant1 : Constant  Value=0
  brake : Outport  InitialOutput=0
  throttle : Outport  Port=2  InitialOutput=0
  wires:
  Constant/1 -> brake/1
  Constant1/1 -> throttle/1

== system ACC_Model/ACC_System/TIS2 ACC action/If Action Subsystem1/If Action Subsystem1/If Action Subsystem1/If Action Subsystem1 ==
  Vp : Inport
  rd : Inport  Port=2
  e [m] : Inport  Port=3
  Action Port : ActionPort  PropagateVarSize=During execution  ActionType=else
  Abs : Abs
  Constant1 : Constant  Value=0
  Constant2 : Constant  Value=LowSpeedActv
  Constant3 : Constant  Value=0
  Divide : Product  Inputs=*/
  Gain : Gain  Gain=3.6
  Gain1 : Gain  Gain=0.5
  Math Function : Math  Operator=square  SaturateOnIntegerOverflow=on
  Relational Operator : RelationalOperator  Operator=<  OutDataTypeStr=boolean
  Saturation1 : Saturate  UpperLimit=inf  LowerLimit=0.02
  Switch : Switch  Criteria=u2 > Threshold
  throttle : Outport  InitialOutput=0
  brake : Outport  Port=2  InitialOutput=0
  wires:
  Constant1/1 -> throttle/1
  Vp/1 -> Gain/1
  Gain/1 -> Relational Operator/1
  Constant2/1 -> Relational Operator/2
  Relational Operator/1 -> Switch/2
  Gain1/1 -> Switch/1
  Constant3/1 -> Switch/3
  rd/1 -> Math Function/1
  Divide/1 -> Gain1/1
  Math Function/1 -> Divide/1
  Abs/1 -> Saturation1/1
  Saturation1/1 -> Divide/2
  e [m]/1 -> Abs/1
  Switch/1 -> brake/1

== system ACC_Model/ACC_System/TIS2 ACC action/Stop & Go/If Action Subsystem/If Action Subsystem/If Action Subsystem ==
  rd : Inport
  e [m] : Inport  Port=2
  dis : Inport  Port=3
  stand : Inport  Port=4
  Action Port : ActionPort  PropagateVarSize=During execution  ActionType=then
  Abs : Abs
  Add : Sum  Inputs=+-
  Bias : Bias  Bias=1
  Constant : Constant  Value=0
  Constant1 : Constant  Value=BrakeMax
  Divide : Product  Inputs=*/
  Gain : Gain  Gain=0.5
  Gain1 : Gain  Gain=J_xx/Qfac/Rw
  Math Function : Math  Operator=square  SaturateOnIntegerOverflow=on
  Saturation : Saturate  UpperLimit=BrakeMax  LowerLimit=0
  Saturation1 : Saturate  UpperLimit=inf  LowerLimit=0.02
  Switch : Switch  Criteria=u2 > Threshold
  brake : Outport  InitialOutput=0
  throttle : Outport  Port=2  InitialOutput=0
  wires:
  rd/1 -> Math Function/1
  Divide/1 -> Gain/1
  Math Function/1 -> Divide/1
  Abs/1 -> Saturation1/1
  Saturation1/1 -> Divide/2
  e [m]/1 -> Abs/1
  Constant/1 -> throttle/1
  Gain/1 -> Saturation/1
  Gain1/1 -> brake/1
  Switch/1 -> Gain1/1
  dis/1 -> Bias/1
  stand/1 -> Add/2
  Add/1 -> Switch/2
  Saturation/1 -> Switch/1
  Constant1/1 -> Switch/3
  Bias/1 -> Add/1
